simulink model "sampleModel293"  (R2021b)
settings: Solver=VariableStepAuto  StartTime=0.0  StopTime=10.0  RelTol=1e-3
libraries: simulink x5, slpidlib x1
settings Model: Creator=user  LastModifiedBy=user

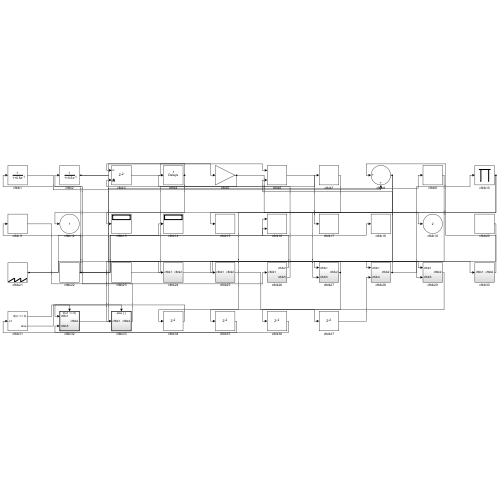
[thumbnail: Simulink's stored preview of the top-level diagram]
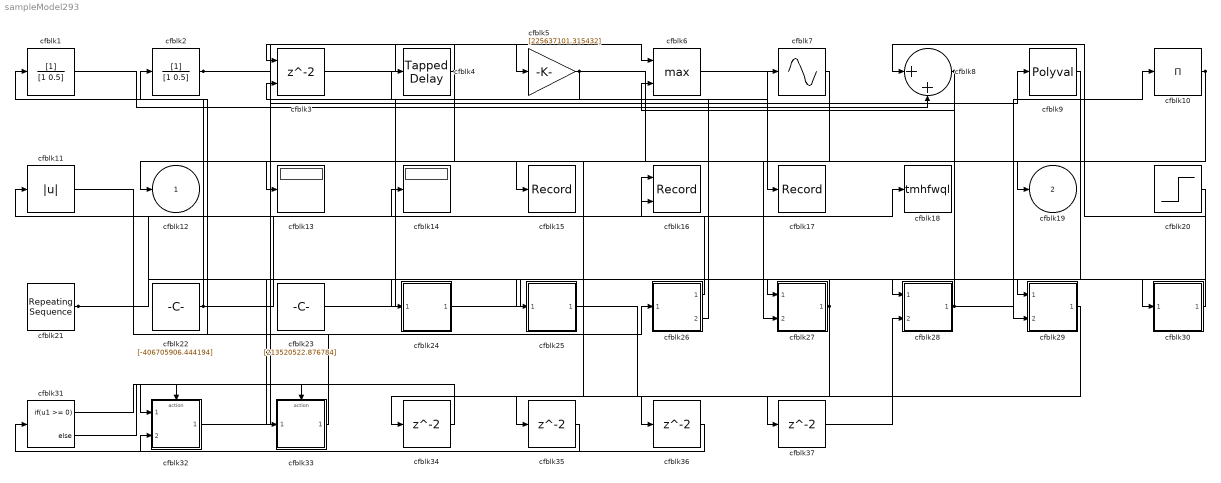
== system sampleModel293 ==
  cfblk1 : DiscreteFilter  SampleTime=1
  cfblk10 : Product  Inputs=*
  cfblk11 : Abs
  cfblk13 : Display
  cfblk14 : Display
  cfblk15 : Record  FileSettingsInternal="{\"entries\":[{\"content\":{\"excelSettings\":{\"content\":{},\"type\":\"Streamout.ExcelSettings\"}},\"type\":\"Streamout.FileSettingStorage\",\"uuid\":\"d99c99a4-b87d-4c9a-a0ee-2737cad6d531\"}],\"packageUris\":[\"http://schema.mathworks.com/mf0/streamout_blocks/R2020a\"],\"version\":\"1.0\"}"  SignalsInternal="{\"entries\":[{\"content\":{\"signals\":[{\"content\":{\"blockPath\":[\"sampleModel293/cfblk15\"],\"channel\":[],\"dimensions\":[1],\"domain\":\"sampleModel293/cfblk15\",\"lineColor\":\"#4dbeee\",\"plots\":[1],\"port\":1,\"sid\":[\"\"],\"signalID\":12562,\"signalName\":\"cfblk7\"},\"type\":\"RecordBlkView.Signal\",\"uuid\":\"48429913-c397-4290-9126-6c6b1df1a7ac\"}]},\"type\":\"RecordBlkView.InputSignals\",\"uuid\":\"9e09da34-561e-4f73-b899-3124a1045019\"}],\"packageUris\":[\"http://schema.mathworks.com/mf0/streamout_blocks/R2020a\"],\"version\":\"1.0\"}"  VisualizationBindings="{\"sparklinesplugin\":{\"info\":[{\"bindingParametersList\":[],\"subplotID\":1}]}}"
  cfblk16 : Record  FileSettingsInternal="{\"entries\":[{\"content\":{\"excelSettings\":{\"content\":{},\"type\":\"Streamout.ExcelSettings\"}},\"type\":\"Streamout.FileSettingStorage\",\"uuid\":\"3b933d8f-505a-45fe-b96f-f71fd841957d\"}],\"packageUris\":[\"http://schema.mathworks.com/mf0/streamout_blocks/R2020a\"],\"version\":\"1.0\"}"  Layout=[1 1]  SignalsInternal="{\"entries\":[{\"content\":{\"signals\":[{\"content\":{\"blockPath\":[\"sampleModel293/cfblk16\"],\"channel\":[],\"dimensions\":[1],\"domain\":\"sampleModel293/cfblk16\",\"lineColor\":\"#a2142f\",\"plots\":[1],\"port\":1,\"sid\":[\"\"],\"signalID\":12550,\"signalName\":\"cfblk26:1\"},\"type\":\"RecordBlkView.Signal\",\"uuid\":\"529dc456-7e45-40f8-804c-43e6a70f2fd8\"},{\"content\":{\"blockPath\":[\"sampleModel293/cfblk16\"],\"channel\":[],\"dimensions\":[1],\"domain\":\"sampleModel293/cfblk16\",\"lineColor\":\"#139fff\",\"plots\":[1],\"port\":2,\"sid\":[\"\"],\"signalID\":12554,\"signalName\":\"cfblk22\"},\"type\":\"RecordBlkView.Signal\",\"uuid\":\"f8dc5db9-cc11-475f-aef1-cb1c0af03a15\"}]},\"type\":\"RecordBlkView.InputSignals\",\"uuid\":\"848a2be6-8bea-4c02-91a3-5ec32db7cc8c\"}],\"packageUris\":[\"http://schema.mathworks.com/mf0/streamout_blocks/R2020a\"],\"version\":\"1.0\"}"  VisualizationBindings="{\"xyplotplugin\":{\"info\":[{\"series\":[{\"bindingParametersList\":[{\"parameter\":\"X-Axis\",\"signalID\":12550,\"signalName\":\"cfblk26:1\"},{\"parameter\":\"Y-Axis\",\"signalID\":12554,\"signalName\":\"cfblk22\"}],\"seriesID\":5117}],\"subplotID\":1}]}}"  CompatibilityTag=XY
  cfblk17 : Record  FileSettingsInternal="{\"entries\":[{\"content\":{\"excelSettings\":{\"content\":{},\"type\":\"Streamout.ExcelSettings\"}},\"type\":\"Streamout.FileSettingStorage\",\"uuid\":\"426f14e6-c4e2-46f0-a989-04dd5aec360d\"}],\"packageUris\":[\"http://schema.mathworks.com/mf0/streamout_blocks/R2020a\"],\"version\":\"1.0\"}"  SignalsInternal="{\"entries\":[{\"content\":{\"signals\":[{\"content\":{\"blockPath\":[\"sampleModel293/cfblk17\"],\"channel\":[],\"dimensions\":[1],\"domain\":\"sampleModel293/cfblk17\",\"lineColor\":\"#77ac30\",\"plots\":[1],\"port\":1,\"sid\":[\"\"],\"signalID\":12558,\"signalName\":\"cfblk6\"},\"type\":\"RecordBlkView.Signal\",\"uuid\":\"4d9e3a2d-1e89-4a65-9dbc-802b2b58537e\"}]},\"type\":\"RecordBlkView.InputSignals\",\"uuid\":\"0fd9211e-f2df-46b2-9a81-9eb1214fc9d5\"}],\"packageUris\":[\"http://schema.mathworks.com/mf0/streamout_blocks/R2020a\"],\"version\":\"1.0\"}"  VisualizationBindings="{\"sparklinesplugin\":{\"info\":[{\"bindingParametersList\":[],\"subplotID\":1}]}}"
  cfblk18 : ToWorkspace  VariableName=tmhfwql  SaveFormat=Timeseries  SampleTime=-1
  cfblk2 : DiscreteFilter  SampleTime=1
  cfblk20 : Step  Time=[48.000000]  Before=[-789311183.428134]  After=[-255497767.535754]  SampleTime=0
  cfblk21 : simulink/Sources/Repeating Sequence  rep_seq_t=[0 2]  rep_seq_y=[-608357566.331030, -488365164.307764]
  cfblk22 : Constant  Value=[-406705906.444194]  SampleTime=1
  cfblk23 : Constant  Value=[213520522.876784]  SampleTime=1
  cfblk24 : Subsystem
  cfblk25 : Subsystem
  cfblk26 : Subsystem
  cfblk27 : Subsystem
  cfblk28 : Subsystem
  cfblk29 : Subsystem
  cfblk3 : Delay  ShowEnablePort=on  SampleTime=1
      settings: InputPortMap=u0,e6
  cfblk30 : Subsystem
  cfblk31 : If  IfExpression=u1 >= 0  SampleTime=1
  cfblk32 : Subsystem  TreatAsAtomicUnit=on
  cfblk33 : Subsystem  TreatAsAtomicUnit=on
  cfblk{34..37} (4 alike) : Delay  SampleTime=1
  cfblk4 : simulink/Discrete/Tapped Delay  vinit=0.0  samptime=-1  NumDelays=1  DelayOrder=Oldest  includeCurrent=off
  cfblk5 : Gain  Gain=[225637101.315432]
  cfblk6 : MinMax  Function=max  Inputs=2
  cfblk7 : Sin  TimeSource=Use external signal  SampleTime=0
  cfblk8 : Sum  Inputs=|++
  cfblk9 : Polyval  Coefs=[ +2.081618890e-019, -1.441693666e-014, +4.719686976e-010, -8.536869453e-006, +1.621573104e-001, -8.087801117e+001 ]
  cfblk12 : Outport
  cfblk19 : Outport  Port=2
  wires:
  cfblk3/1 -> cfblk6/1
  cfblk24/1(cfblk2) -> cfblk30/1(cfblk1)
  cfblk8/1 -> cfblk12/1, cfblk33/1(cfblk1)
  cfblk26/1(cfblk2) -> cfblk16/1
  cfblk11/1 -> cfblk26/1(cfblk1)
  cfblk32/1(cfblk2) -> cfblk9/1
  cfblk30/1(cfblk2) -> cfblk8/1
  cfblk33/1(cfblk2) -> cfblk2/1
  cfblk9/1 -> cfblk28/1(cfblk1)
  cfblk22/1 -> cfblk29/1(cfblk1), cfblk1/1, cfblk18/1, cfblk11/1, cfblk16/2
  cfblk10/1 -> cfblk27/2(cfblk5), cfblk35/1
  cfblk5/1 -> cfblk19/1, cfblk3/2
  cfblk6/1 -> cfblk17/1
  cfblk23/1 -> cfblk7/1
  cfblk2/1 -> cfblk29/2(cfblk5), cfblk5/1
  cfblk1/1 -> cfblk8/2
  cfblk7/1 -> cfblk15/1
  cfblk20/1 -> cfblk27/1(cfblk1)
  cfblk28/1(cfblk2) -> cfblk6/2, cfblk10/1
  cfblk4/1 -> cfblk13/1, cfblk3/1
  cfblk21/1 -> cfblk24/1(cfblk1), cfblk14/1
  cfblk27/1(cfblk2) -> cfblk25/1(cfblk1), cfblk36/1
  cfblk26/2(cfblk5) -> cfblk4/1
  cfblk31/1 -> cfblk32/Action
  cfblk31/2 -> cfblk33/Action
  cfblk29/1(cfblk2) -> cfblk34/1
  cfblk34/1 -> cfblk32/1(cfblk1)
  cfblk35/1 -> cfblk31/1
  cfblk36/1 -> cfblk32/2(cfblk5)
  cfblk25/1(cfblk2) -> cfblk37/1
  cfblk37/1 -> cfblk28/2(cfblk4)

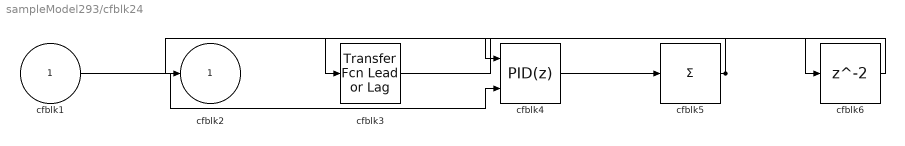
== system sampleModel293/cfblk24 ==
  cfblk1 : Inport
  cfblk3 : simulink/Discrete/Transfer Fcn Lead or Lag  PoleZ=0.95  ZeroZ=0.75  ICPrevOutput=0.0  ICPrevInput=0.0  DoSatur=off
      settings: SourceProductBaseCode=SL
  cfblk4 : slpidlib/PID Controller (2DOF)  Controller=PID  Form=Parallel  TimeDomain=Discrete-time  UseExternalTs=off  SampleTime=1  IntegratorMethod=Forward Euler  FilterMethod=Forward Euler  ControllerParametersSource=internal  P=1  I=1  D=0  UseFilter=on  N=100  b=1  c=1  TunerSelectOption=Transfer Function Based (PID Tuner App)  InitialConditionSource=internal  InitialConditionForIntegrator=0  InitialConditionForFilter=0  DifferentiatorICPrevScaledInput=0  ExternalReset=none  TrackingMode=off  Kt=1  LimitOutput=off  SatLimitsSource=internal  UpperSaturationLimit=inf  LowerSaturationLimit=-inf  LinearizeAsGain=off  AntiWindupMode=none  Kb=1  POutMin=[]  POutMax=[]  IOutMin=[]  IOutMax=[]  DOutMin=[]  DOutMax=[]  NOutMin=[]  NOutMax=[]  bOutMin=[]  bOutMax=[]  cOutMin=[]  cOutMax=[]  SumOutMin=[]  SumOutMax=[]  SaturationOutMin=[]  SaturationOutMax=[]  PParamMin=[]  PParamMax=[]  IParamMin=[]  IParamMax=[]  DParamMin=[]  DParamMax=[]  NParamMin=[]  NParamMax=[]  bParamMin=[]  bParamMax=[]  cParamMin=[]  cParamMax=[]  KbParamMin=[]  KbParamMax=[]  KtParamMin=[]  KtParamMax=[]  KbOutMin=[]  KbOutMax=[]  KtOutMin=[]  KtOutMax=[]  IntegratorOutMin=[]  IntegratorOutMax=[]  FilterOutMin=[]  FilterOutMax=[]  SumI1OutMin=[]  SumI1OutMax=[]  SumI2OutMin=[]  SumI2OutMax=[]  SumI3OutMin=[]  SumI3OutMax=[]  SumI4OutMin=[]  SumI4OutMax=[]  SumDOutMin=[]  SumDOutMax=[]  Sum1OutMin=[]  Sum1OutMax=[]  Sum2OutMin=[]  Sum2OutMax=[]  Sum3OutMin=[]  Sum3OutMax=[]  DifferentiatorOutMin=[]  DifferentiatorOutMax=[]  FilterDiffOutCoefMin=[]  FilterDiffOutCoefMax=[]  ReciprocalOutMin=[]  ReciprocalOutMax=[]  SumDenOutMin=[]  SumDenOutMax=[]  SumNumOutMin=[]  SumNumOutMax=[]  DivideOutMin=[]  DivideOutMax=[]  UdiffTsProdOutMin=[]  UdiffTsProdOutMax=[]  NTsProdOutMin=[]  NTsProdOutMax=[]  UintegralTsProdOutMin=[]  UintegralTsProdOutMax=[]  UngainTsProdOutMin=[]  UngainTsProdOutMax=[]  IntegratorContinuousStateAttributes=''  IntegratorStateMustResolveToSignalObject=off  IntegratorRTWStateStorageClass=Auto  FilterContinuousStateAttributes=''  FilterStateMustResolveToSignalObject=off  FilterRTWStateStorageClass=Auto  ParallelPVariant=InternalParameters  IdealPVariant=Disabled  IVariant=InternalParameters  DVariant=InternalParameters  bVariant=InternalParameters  cVariant=InternalParameters  IntegratorVariant=Discrete  SatVariant=Disabled  AWVariant=Passthrough  PCopyVariant=Disabled  TRVariant=Disabled  FdbkBlocksVariant=Forward  IdealPFdbkVariant=Disabled  SatFdbkVariant=Disabled  DerivativeFilterVariant=ForwardEulerFilter  NVariant=InternalParameters  NCopyVariant=Disabled  FilterICVariant=InternalICsFilter  IntegratorICVariant=InternalICs  ExternalResetVariant=Disabled  TRSumVariant=Passthrough  SumFdbkVariant=Disabled  SumVariant=Sum_PID  TsampFilterVariant=InternalTs  TsampNgainVariant=Passthrough  TsampIntegralVariant=Passthrough  ExternalSaturationOutDataTypeStr=Inherit: Same as second input
      settings: SourceProductBaseCode=SL
  cfblk5 : Sum  Inputs=+
  cfblk6 : Delay  SampleTime=1
  cfblk2 : Outport
  wires:
  cfblk4/1 -> cfblk5/1
  cfblk5/1 -> cfblk3/1, cfblk2/1
  cfblk1/1 -> cfblk4/2
  cfblk3/1 -> cfblk6/1
  cfblk6/1 -> cfblk4/1

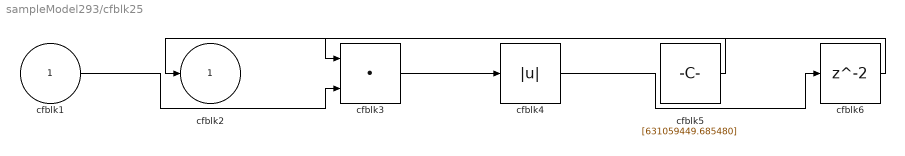
== system sampleModel293/cfblk25 ==
  cfblk1 : Inport
  cfblk3 : DotProduct  InputSameDT=on  OutDataTypeStr=Inherit: Inherit via internal rule
  cfblk4 : Abs
  cfblk5 : Constant  Value=[631059449.685480]  SampleTime=1
  cfblk6 : Delay  SampleTime=1
  cfblk2 : Outport
  wires:
  cfblk5/1 -> cfblk2/1
  cfblk1/1 -> cfblk3/2
  cfblk3/1 -> cfblk4/1
  cfblk4/1 -> cfblk6/1
  cfblk6/1 -> cfblk3/1

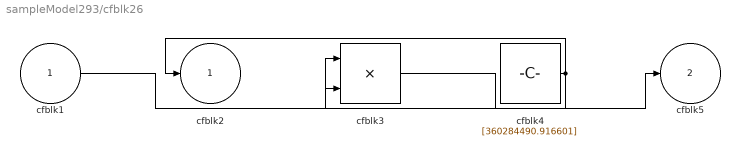
== system sampleModel293/cfblk26 ==
  cfblk1 : Inport
  cfblk3 : Product
  cfblk4 : Constant  Value=[360284490.916601]  SampleTime=1
  cfblk2 : Outport
  cfblk5 : Outport  Port=2
  wires:
  cfblk4/1 -> cfblk2/1, cfblk3/2
  cfblk1/1 -> cfblk3/1
  cfblk3/1 -> cfblk5/1

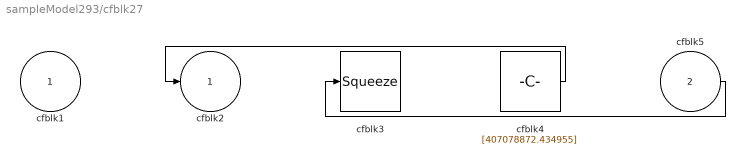
== system sampleModel293/cfblk27 ==
  cfblk1 : Inport
  cfblk5 : Inport  Port=2
  cfblk3 : Squeeze
  cfblk4 : Constant  Value=[407078872.434955]  SampleTime=1
  cfblk2 : Outport
  wires:
  cfblk4/1 -> cfblk2/1
  cfblk5/1 -> cfblk3/1

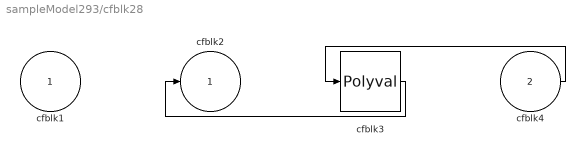
== system sampleModel293/cfblk28 ==
  cfblk1 : Inport
  cfblk4 : Inport  Port=2
  cfblk3 : Polyval  Coefs=[ +2.081618890e-019, -1.441693666e-014, +4.719686976e-010, -8.536869453e-006, +1.621573104e-001, -8.087801117e+001 ]
  cfblk2 : Outport
  wires:
  cfblk4/1 -> cfblk3/1
  cfblk3/1 -> cfblk2/1

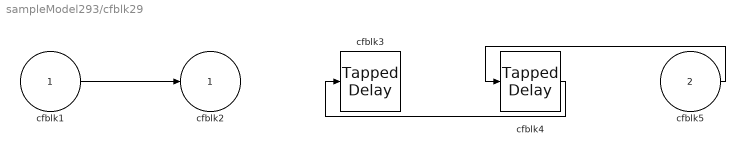
== system sampleModel293/cfblk29 ==
  cfblk1 : Inport
  cfblk5 : Inport  Port=2
  cfblk3 : simulink/Discrete/Tapped Delay  vinit=0.0  samptime=-1  NumDelays=1  DelayOrder=Oldest  includeCurrent=off
  cfblk4 : simulink/Discrete/Tapped Delay  vinit=0.0  samptime=-1  NumDelays=1  DelayOrder=Oldest  includeCurrent=off
  cfblk2 : Outport
  wires:
  cfblk5/1 -> cfblk4/1
  cfblk1/1 -> cfblk2/1
  cfblk4/1 -> cfblk3/1

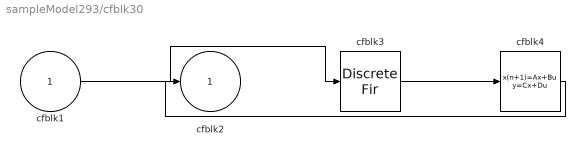
== system sampleModel293/cfblk30 ==
  cfblk1 : Inport
  cfblk3 : DiscreteFir  SampleTime=1
  cfblk4 : DiscreteStateSpace
  cfblk2 : Outport
  wires:
  cfblk1/1 -> cfblk3/1
  cfblk4/1 -> cfblk2/1
  cfblk3/1 -> cfblk4/1

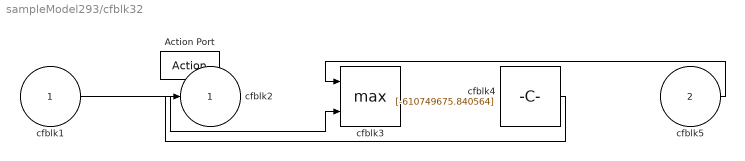
== system sampleModel293/cfblk32 ==
  cfblk1 : Inport
  cfblk5 : Inport  Port=2
  Action Port : ActionPort  ActionPortLabel=if(u1 >= 0)
  cfblk3 : MinMax  Function=max  Inputs=2
  cfblk4 : Constant  Value=[-610749675.840564]  SampleTime=1
  cfblk2 : Outport
  wires:
  cfblk5/1 -> cfblk3/1
  cfblk1/1 -> cfblk3/2
  cfblk4/1 -> cfblk2/1

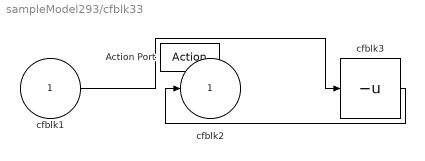
== system sampleModel293/cfblk33 ==
  cfblk1 : Inport
  Action Port : ActionPort  ActionPortLabel=else
  cfblk3 : UnaryMinus
  cfblk2 : Outport
  wires:
  cfblk3/1 -> cfblk2/1
  cfblk1/1 -> cfblk3/1
